simulink model "Rocketmodel"  (R2024b)
settings: Solver=FixedStepDiscrete  StartTime=0.0  StopTime=20  FixedStep=0.001  RelTol=1e-3
values from neighbouring files (symbols this model uses):
  Euler0 = [0 0 -3]/57.3    [Trajectory_Optimization.m]
  Omega0 = [0 0 0]/57.3    [Trajectory_Optimization.m]
  R0 = [36 748 0]    [Trajectory_Optimization.m]
  V0 = [-8.6 -69.6 0]    [Trajectory_Optimization.m]
undefined symbols (not defined in the file or in its folder): den_Engine, den_GZ, den_SF, DiscIntNeverNeededParam, dspblkCoreblockFVToolHelper, Euler, gcbh, num_Engine, num_GZ, num_SF, R, Tc, Ts
libraries: simulink x2
settings Model: Creator=Administrator  LastModifiedBy=Administrator
settings SolverCC: AlgebraicLoopSolver=TrustRegion
settings DebuggingCC: ArithmeticOperatorsInVariantConditions=warning
settings SFSimCC: CustomCodeUndefinedFunction=UseInterfaceOnly
settings RTWCC: GPUComputeCapability=3.5

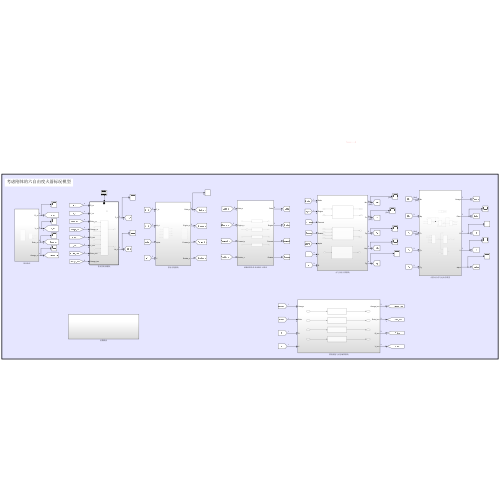
[thumbnail: Simulink's stored preview of the top-level diagram]
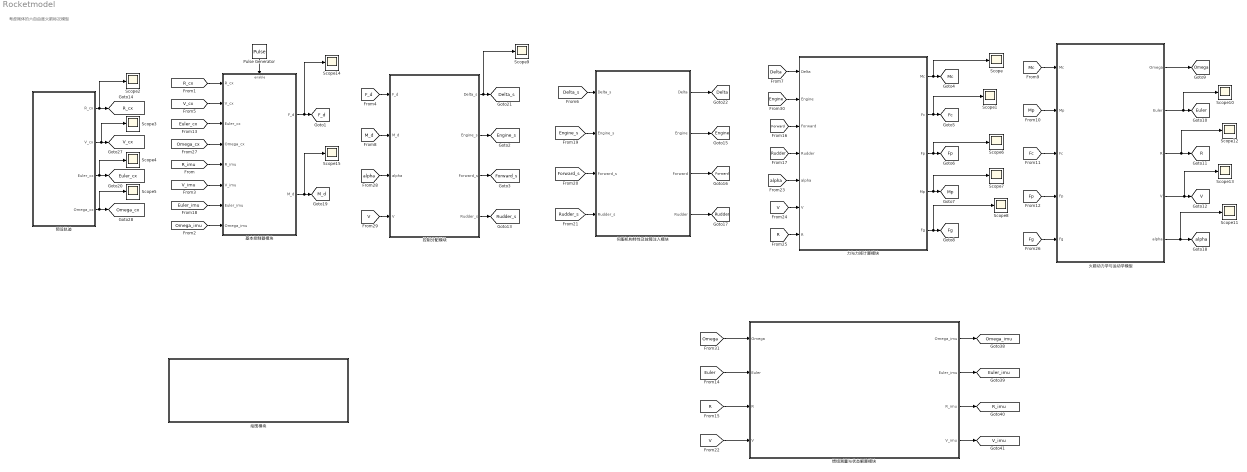
== system Rocketmodel ==
  note: 考虑刚体的六自由度火箭标况模型
  Pulse Generator : DiscretePulseGenerator  Period=Tc/Ts  SampleTime=-1
  Scope{,1..15} (16 alike) : Scope
  伺服机构特性及故障注入模块 : Subsystem
  力与力矩计算模块 : Subsystem
  基本控制器模块 : Subsystem  TreatAsAtomicUnit=on
  惯组测量与状态解算模块 : Subsystem
  控制分配模块 : Subsystem
  火箭动力学与运动学模型 : Subsystem
  绘图模块 : Subsystem
  预设轨迹 : Subsystem
  tag scope: Delta=global, Delta_s=global, Engine=global, Engine_s=global, Euler=global, Euler_cx=global, Euler_imu=global, F_d=global, Fc=global, Fg=global, Forward=global, Forward_s=global, Fp=global, M_d=global, Mc=global, Mp=global, Omega=global, Omega_cx=global, Omega_imu=global, R=global, R_cx=global, R_imu=global, Rudder=global, Rudder_s=global, V=global, V_cx=global, V_imu=global, alpha=global
  wires:
  基本控制器模块/2(M_d) -> Scope15/1, [M_d]
  [Delta_s] -> 伺服机构特性及故障注入模块/1(Delta_s)
  [R_cx] -> 基本控制器模块/1(R_cx)
  Pulse Generator/1 -> 基本控制器模块/Enable
  [R_imu] -> 基本控制器模块/5(R_imu)
  [Euler_imu] -> 基本控制器模块/7(Euler_imu)
  [Omega] -> 惯组测量与状态解算模块/1(Omega)
  惯组测量与状态解算模块/1(Omega_imu) -> [Omega_imu]
  惯组测量与状态解算模块/2(Euler_imu) -> [Euler_imu]
  惯组测量与状态解算模块/3(R_imu) -> [R_imu]
  [Omega_imu] -> 基本控制器模块/8(Omega_imu)
  [V_imu] -> 基本控制器模块/6(V_imu)
  基本控制器模块/1(F_d) -> Scope14/1, [F_d]
  伺服机构特性及故障注入模块/1(Delta) -> [Delta]
  [Engine_s] -> 伺服机构特性及故障注入模块/2(Engine_s)
  [Forward_s] -> 伺服机构特性及故障注入模块/3(Forward_s)
  [Rudder_s] -> 伺服机构特性及故障注入模块/4(Rudder_s)
  伺服机构特性及故障注入模块/4(Rudder) -> [Rudder]
  伺服机构特性及故障注入模块/3(Forward) -> [Forward]
  伺服机构特性及故障注入模块/2(Engine) -> [Engine]
  [Delta] -> 力与力矩计算模块/1(Delta)
  [Engine] -> 力与力矩计算模块/2(Engine)
  [Forward] -> 力与力矩计算模块/3(Forward)
  [Rudder] -> 力与力矩计算模块/4(Rudder)
  力与力矩计算模块/1(Mc) -> Scope/1, [Mc]
  力与力矩计算模块/5(Fg) -> Scope8/1, [Fg]
  力与力矩计算模块/4(Mp) -> Scope7/1, [Mp]
  力与力矩计算模块/3(Fp) -> Scope6/1, [Fp]
  力与力矩计算模块/2(Fc) -> Scope1/1, [Fc]
  [Mc] -> 火箭动力学与运动学模型/1(Mc)
  [Fc] -> 火箭动力学与运动学模型/3(Fc)
  [Fp] -> 火箭动力学与运动学模型/4(Fp)
  [Mp] -> 火箭动力学与运动学模型/2(Mp)
  火箭动力学与运动学模型/1(Omega) -> [Omega]
  火箭动力学与运动学模型/2(Euler) -> Scope10/1, [Euler]
  火箭动力学与运动学模型/3(R) -> Scope12/1, [R]
  火箭动力学与运动学模型/4(V) -> Scope13/1, [V]
  火箭动力学与运动学模型/5(alpha) -> Scope11/1, [alpha]
  [Euler] -> 惯组测量与状态解算模块/2(Euler)
  [R] -> 惯组测量与状态解算模块/3(R)
  [V] -> 惯组测量与状态解算模块/4(V)
  惯组测量与状态解算模块/4(V_imu) -> [V_imu]
  [V] -> 力与力矩计算模块/6(V)
  [R] -> 力与力矩计算模块/7(R)
  [Fg] -> 火箭动力学与运动学模型/5(Fg)
  ? -> ?
  预设轨迹/1(R_cx) -> [R_cx], Scope2/1
  预设轨迹/3(Euler_cx) -> Scope4/1, [Euler_cx]
  预设轨迹/2(V_cx) -> Scope3/1, [V_cx]
  预设轨迹/4(Omega_cx) -> Scope5/1, [Omega_cx]
  [Omega_cx] -> 基本控制器模块/4(Omega_cx)
  [Euler_cx] -> 基本控制器模块/3(Euler_cx)
  [V_cx] -> 基本控制器模块/2(V_cx)
  [alpha] -> 力与力矩计算模块/5(alpha)
  [M_d] -> 控制分配模块/2(M_d)
  控制分配模块/3(Forward_s) -> [Forward_s]
  [F_d] -> 控制分配模块/1(F_d)
  控制分配模块/2(Engine_s) -> [Engine_s]
  控制分配模块/1(Delta_s) -> Scope9/1, [Delta_s]
  控制分配模块/4(Rudder_s) -> [Rudder_s]
  [alpha] -> 控制分配模块/3(alpha)
  [V] -> 控制分配模块/4(V)

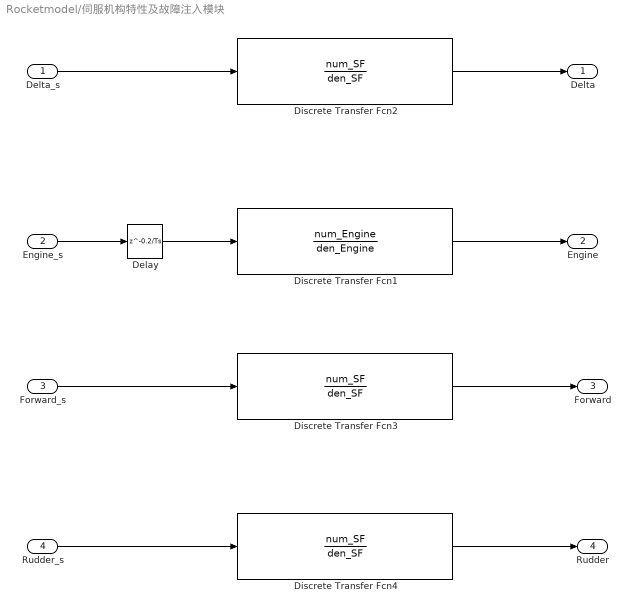
== system Rocketmodel/伺服机构特性及故障注入模块 ==
  Delta_s : Inport
  Engine_s : Inport  Port=2
  Forward_s : Inport  Port=3
  Rudder_s : Inport  Port=4
  Delay : Delay  DelayLength=0.2/Ts  InitialCondition=0
  Discrete Transfer Fcn1 : DiscreteTransferFcn  LoadFcn=dspblkCoreblockFVToolHelper(gcbh,'load');  Numerator=num_Engine  Denominator=den_Engine
      settings: CopyFcn=dspblkCoreblockFVToolHelper(gcbh,'copy');  DeleteFcn=dspblkCoreblockFVToolHelper(gcbh,'close');  ModelCloseFcn=dspblkCoreblockFVToolHelper(gcbh,'close');  PreSaveFcn=dspblkCoreblockFVToolHelper(gcbh,'presave');  PostSaveFcn=dspblkCoreblockFVToolHelper(gcbh,'postsave');  CloseFcn=dspblkCoreblockFVToolHelper(gcbh,'close');
  Discrete Transfer Fcn2 : DiscreteTransferFcn  LoadFcn=dspblkCoreblockFVToolHelper(gcbh,'load');  Numerator=num_SF  Denominator=den_SF
      settings: CopyFcn=dspblkCoreblockFVToolHelper(gcbh,'copy');  DeleteFcn=dspblkCoreblockFVToolHelper(gcbh,'close');  ModelCloseFcn=dspblkCoreblockFVToolHelper(gcbh,'close');  PreSaveFcn=dspblkCoreblockFVToolHelper(gcbh,'presave');  PostSaveFcn=dspblkCoreblockFVToolHelper(gcbh,'postsave');  CloseFcn=dspblkCoreblockFVToolHelper(gcbh,'close');
  Discrete Transfer Fcn3 : DiscreteTransferFcn  LoadFcn=dspblkCoreblockFVToolHelper(gcbh,'load');  Numerator=num_SF  Denominator=den_SF
      settings: CopyFcn=dspblkCoreblockFVToolHelper(gcbh,'copy');  DeleteFcn=dspblkCoreblockFVToolHelper(gcbh,'close');  ModelCloseFcn=dspblkCoreblockFVToolHelper(gcbh,'close');  PreSaveFcn=dspblkCoreblockFVToolHelper(gcbh,'presave');  PostSaveFcn=dspblkCoreblockFVToolHelper(gcbh,'postsave');  CloseFcn=dspblkCoreblockFVToolHelper(gcbh,'close');
  Discrete Transfer Fcn4 : DiscreteTransferFcn  LoadFcn=dspblkCoreblockFVToolHelper(gcbh,'load');  Numerator=num_SF  Denominator=den_SF
      settings: CopyFcn=dspblkCoreblockFVToolHelper(gcbh,'copy');  DeleteFcn=dspblkCoreblockFVToolHelper(gcbh,'close');  ModelCloseFcn=dspblkCoreblockFVToolHelper(gcbh,'close');  PreSaveFcn=dspblkCoreblockFVToolHelper(gcbh,'presave');  PostSaveFcn=dspblkCoreblockFVToolHelper(gcbh,'postsave');  CloseFcn=dspblkCoreblockFVToolHelper(gcbh,'close');
  Delta : Outport
  Engine : Outport  Port=2
  Forward : Outport  Port=3
  Rudder : Outport  Port=4
  wires:
  Delay/1 -> Discrete Transfer Fcn1/1
  Engine_s/1 -> Delay/1
  Delta_s/1 -> Discrete Transfer Fcn2/1
  Forward_s/1 -> Discrete Transfer Fcn3/1
  Rudder_s/1 -> Discrete Transfer Fcn4/1
  Discrete Transfer Fcn2/1 -> Delta/1
  Discrete Transfer Fcn1/1 -> Engine/1
  Discrete Transfer Fcn3/1 -> Forward/1
  Discrete Transfer Fcn4/1 -> Rudder/1

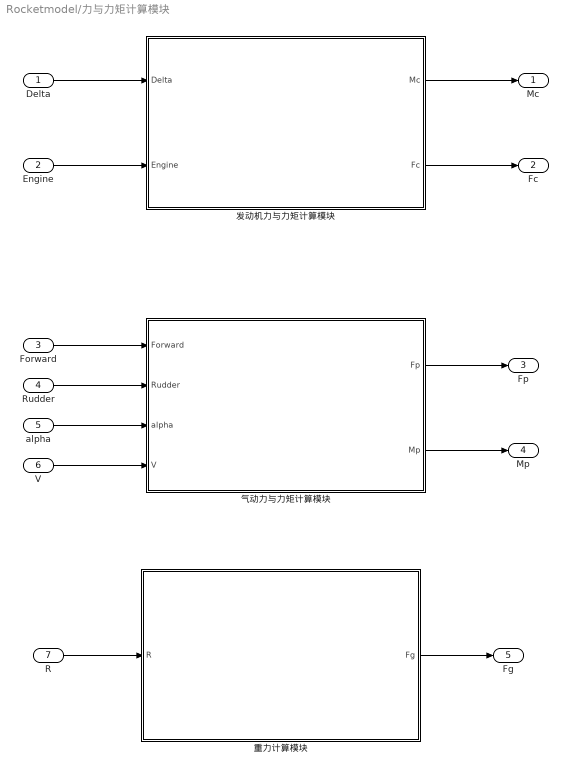
== system Rocketmodel/力与力矩计算模块 ==
  Delta : Inport
  Engine : Inport  Port=2
  Forward : Inport  Port=3
  Rudder : Inport  Port=4
  alpha : Inport  Port=5
  V : Inport  Port=6
  R : Inport  Port=7
  发动机力与力矩计算模块 : Subsystem
  气动力与力矩计算模块 : Subsystem
  重力计算模块 : Subsystem
  Mc : Outport
  Fc : Outport  Port=2
  Fp : Outport  Port=3
  Mp : Outport  Port=4
  Fg : Outport  Port=5
  wires:
  发动机力与力矩计算模块/2(Fc) -> Fc/1
  发动机力与力矩计算模块/1(Mc) -> Mc/1
  Delta/1 -> 发动机力与力矩计算模块/1(Delta)
  Engine/1 -> 发动机力与力矩计算模块/2(Engine)
  Forward/1 -> 气动力与力矩计算模块/1(Forward)
  Rudder/1 -> 气动力与力矩计算模块/2(Rudder)
  alpha/1 -> 气动力与力矩计算模块/3(alpha)
  V/1 -> 气动力与力矩计算模块/4(V)
  气动力与力矩计算模块/2(Mp) -> Mp/1
  气动力与力矩计算模块/1(Fp) -> Fp/1
  R/1 -> 重力计算模块/1(R)
  重力计算模块/1(Fg) -> Fg/1

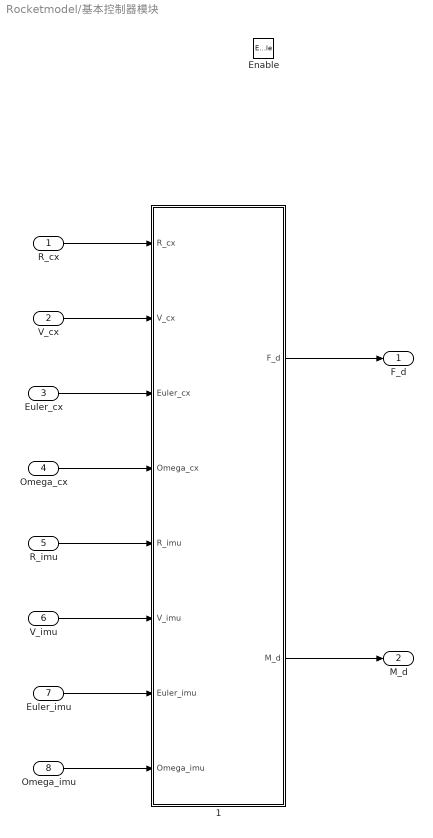
== system Rocketmodel/基本控制器模块 ==
  R_cx : Inport
  V_cx : Inport  Port=2
  Euler_cx : Inport  Port=3
  Omega_cx : Inport  Port=4
  R_imu : Inport  Port=5
  V_imu : Inport  Port=6
  Euler_imu : Inport  Port=7
  Omega_imu : Inport  Port=8
  Enable : EnablePort
  1 : MATLAB Function  TreatAsAtomicUnit=on
  F_d : Outport
  M_d : Outport  Port=2
  wires:
  R_cx/1 -> 1/1(R_cx)
  R_imu/1 -> 1/5(R_imu)
  V_imu/1 -> 1/6(V_imu)
  Euler_imu/1 -> 1/7(Euler_imu)
  Omega_imu/1 -> 1/8(Omega_imu)
  1/1(F_d) -> F_d/1
  V_cx/1 -> 1/2(V_cx)
  Euler_cx/1 -> 1/3(Euler_cx)
  Omega_cx/1 -> 1/4(Omega_cx)
  1/2(M_d) -> M_d/1

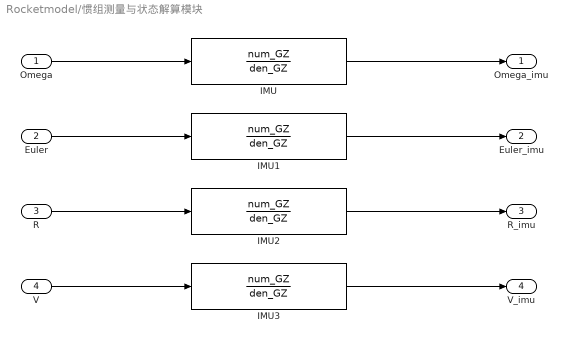
== system Rocketmodel/惯组测量与状态解算模块 ==
  Omega : Inport
  Euler : Inport  Port=2
  R : Inport  Port=3
  V : Inport  Port=4
  IMU{,1..3} (4 alike) : DiscreteTransferFcn  LoadFcn=dspblkCoreblockFVToolHelper(gcbh,'load');  Numerator=num_GZ  Denominator=den_GZ
      settings: CopyFcn=dspblkCoreblockFVToolHelper(gcbh,'copy');  DeleteFcn=dspblkCoreblockFVToolHelper(gcbh,'close');  ModelCloseFcn=dspblkCoreblockFVToolHelper(gcbh,'close');  PreSaveFcn=dspblkCoreblockFVToolHelper(gcbh,'presave');  PostSaveFcn=dspblkCoreblockFVToolHelper(gcbh,'postsave');  CloseFcn=dspblkCoreblockFVToolHelper(gcbh,'close');
  Omega_imu : Outport
  Euler_imu : Outport  Port=2
  R_imu : Outport  Port=3
  V_imu : Outport  Port=4
  wires:
  IMU/1 -> Omega_imu/1
  Omega/1 -> IMU/1
  IMU3/1 -> V_imu/1
  IMU2/1 -> R_imu/1
  IMU1/1 -> Euler_imu/1
  Euler/1 -> IMU1/1
  R/1 -> IMU2/1
  V/1 -> IMU3/1

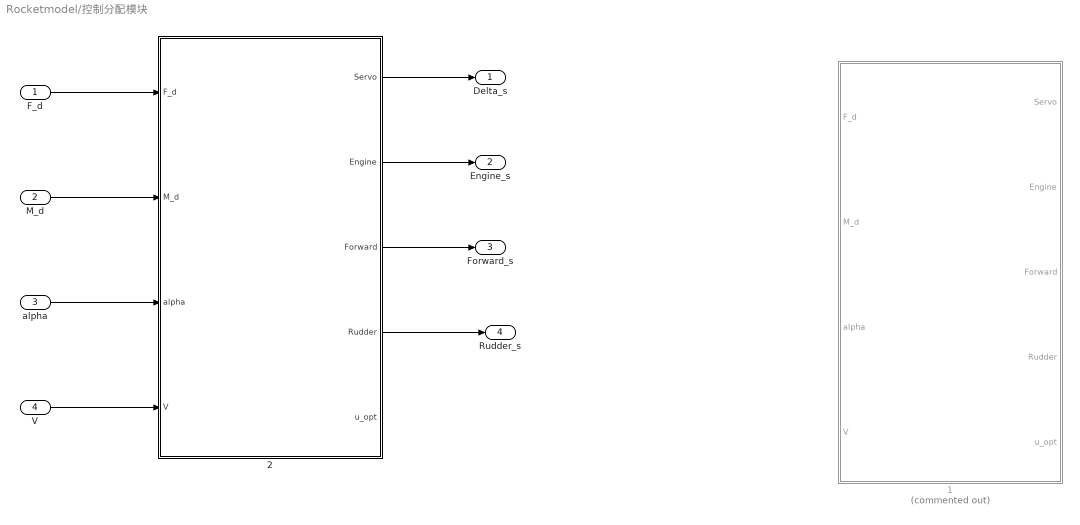
== system Rocketmodel/控制分配模块 ==
  F_d : Inport
  M_d : Inport  Port=2
  alpha : Inport  Port=3
  V : Inport  Port=4
  1 : MATLAB Function  Commented=on  TreatAsAtomicUnit=on
  2 : MATLAB Function  TreatAsAtomicUnit=on
  Delta_s : Outport
  Engine_s : Outport  Port=2
  Forward_s : Outport  Port=3
  Rudder_s : Outport  Port=4
  wires:
  2/1(Servo) -> Delta_s/1
  2/2(Engine) -> Engine_s/1
  2/3(Forward) -> Forward_s/1
  2/4(Rudder) -> Rudder_s/1
  F_d/1 -> 2/1(F_d)
  M_d/1 -> 2/2(M_d)
  alpha/1 -> 2/3(alpha)
  V/1 -> 2/4(V)

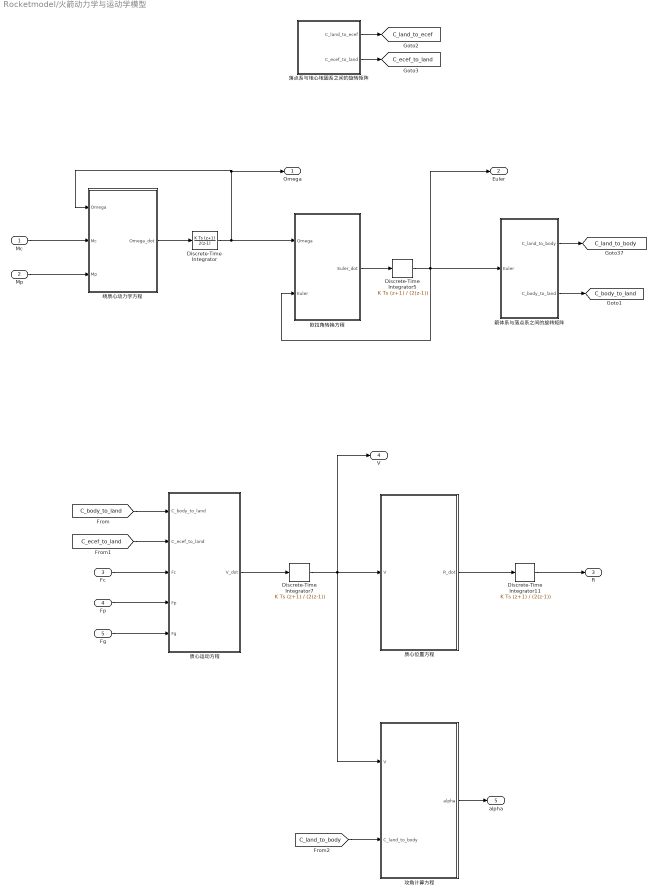
== system Rocketmodel/火箭动力学与运动学模型 ==
  Mc : Inport
  Mp : Inport  Port=2
  Fc : Inport  Port=3
  Fp : Inport  Port=4
  Fg : Inport  Port=5
  Discrete-Time Integrator : DiscreteIntegrator  IntegratorMethod=Integration: Trapezoidal  InitialCondition=Omega0  SampleTime=-1  ICPrevOutput=DiscIntNeverNeededParam  ICPrevScaledInput=DiscIntNeverNeededParam
  Discrete-Time Integrator11 : DiscreteIntegrator  IntegratorMethod=Integration: Trapezoidal  InitialCondition=R0  SampleTime=-1  ICPrevOutput=DiscIntNeverNeededParam  ICPrevScaledInput=DiscIntNeverNeededParam
  Discrete-Time Integrator5 : DiscreteIntegrator  IntegratorMethod=Integration: Trapezoidal  InitialCondition=Euler0  SampleTime=-1  ICPrevOutput=DiscIntNeverNeededParam  ICPrevScaledInput=DiscIntNeverNeededParam
  Discrete-Time Integrator7 : DiscreteIntegrator  IntegratorMethod=Integration: Trapezoidal  InitialCondition=V0  SampleTime=-1  ICPrevOutput=DiscIntNeverNeededParam  ICPrevScaledInput=DiscIntNeverNeededParam
  攻角计算方程 : MATLAB Function  TreatAsAtomicUnit=on
  欧拉角转换方程 : MATLAB Function  TreatAsAtomicUnit=on
  箭体系与落点系之间的旋转矩阵 : MATLAB Function  TreatAsAtomicUnit=on
  绕质心动力学方程 : MATLAB Function  TreatAsAtomicUnit=on
  落点系与地心地固系之间的旋转矩阵 : MATLAB Function  TreatAsAtomicUnit=on
  质心位置方程 : MATLAB Function  TreatAsAtomicUnit=on
  质心运动方程 : MATLAB Function  TreatAsAtomicUnit=on
  Omega : Outport
  Euler : Outport  Port=2
  R : Outport  Port=3
  V : Outport  Port=4
  alpha : Outport  Port=5
  tag scope: C_body_to_land=global, C_ecef_to_land=global, C_land_to_body=global, C_land_to_ecef=global
  wires:
  Fp/1 -> 质心运动方程/4(Fp)
  Mc/1 -> 绕质心动力学方程/2(Mc)
  绕质心动力学方程/1(Omega_dot) -> Discrete-Time Integrator/1
  质心位置方程/1(R_dot) -> Discrete-Time Integrator11/1
  落点系与地心地固系之间的旋转矩阵/2(C_ecef_to_land) -> [C_ecef_to_land]
  质心运动方程/1(V_dot) -> Discrete-Time Integrator7/1
  [C_body_to_land] -> 质心运动方程/1(C_body_to_land)
  Discrete-Time Integrator5/1 -> Euler/1, 箭体系与落点系之间的旋转矩阵/1(Euler), 欧拉角转换方程/2(Euler)
  Mp/1 -> 绕质心动力学方程/3(Mp)
  落点系与地心地固系之间的旋转矩阵/1(C_land_to_ecef) -> [C_land_to_ecef]
  Fg/1 -> 质心运动方程/5(Fg)
  Discrete-Time Integrator7/1 -> 攻角计算方程/1(V), V/1, 质心位置方程/1(V)
  Discrete-Time Integrator/1 -> 欧拉角转换方程/1(Omega), 绕质心动力学方程/1(Omega), Omega/1
  [C_ecef_to_land] -> 质心运动方程/2(C_ecef_to_land)
  箭体系与落点系之间的旋转矩阵/1(C_land_to_body) -> [C_land_to_body]
  Discrete-Time Integrator11/1 -> R/1
  欧拉角转换方程/1(Euler_dot) -> Discrete-Time Integrator5/1
  攻角计算方程/1(alpha) -> alpha/1
  Fc/1 -> 质心运动方程/3(Fc)
  [C_land_to_body] -> 攻角计算方程/2(C_land_to_body)
  箭体系与落点系之间的旋转矩阵/2(C_body_to_land) -> [C_body_to_land]

== system Rocketmodel/绘图模块 ==

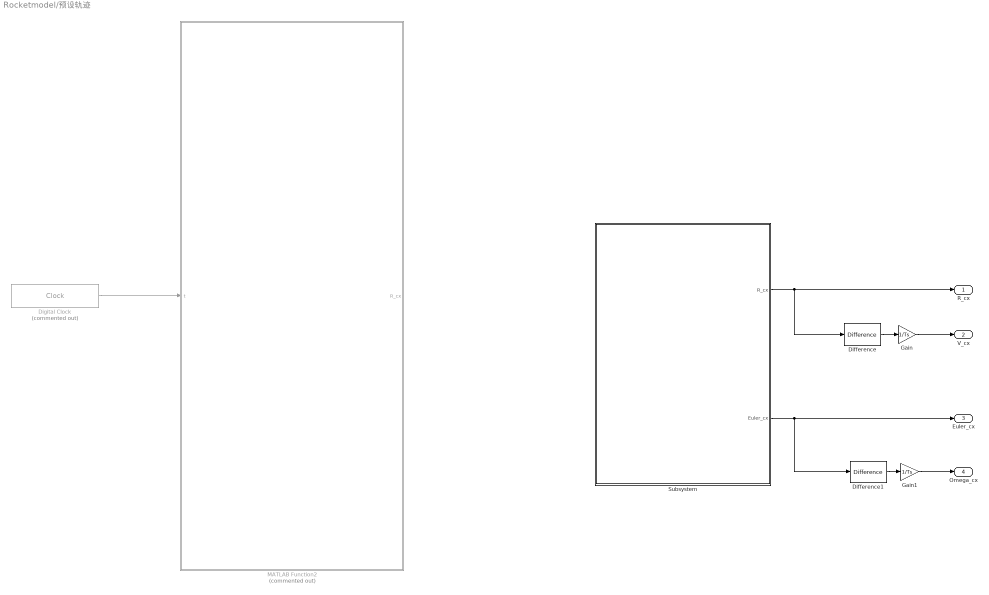
== system Rocketmodel/预设轨迹 ==
  Difference : simulink/Discrete/Difference  ICPrevInput=R(:,1)  OutMin=[]  OutMax=[]  OutDataType=fixdt(1, 16)  OutScaling=2^-10  DoSatur=off
  Difference1 : simulink/Discrete/Difference  ICPrevInput=Euler(:,1)  OutMin=[]  OutMax=[]  OutDataType=fixdt(1, 16)  OutScaling=2^-10  DoSatur=off
  Digital Clock : DigitalClock  Commented=on  SampleTime=Ts
  Gain : Gain  Gain=1/Ts
  Gain1 : Gain  Gain=1/Ts
  MATLAB Function2 : MATLAB Function  Commented=on  TreatAsAtomicUnit=on
  Subsystem : Subsystem
  R_cx : Outport
  V_cx : Outport  Port=2
  Euler_cx : Outport  Port=3
  Omega_cx : Outport  Port=4
  wires:
  Digital Clock/1 -> MATLAB Function2/1(t)
  Difference/1 -> Gain/1
  Difference1/1 -> Gain1/1
  Subsystem/1(R_cx) -> Difference/1, R_cx/1
  Subsystem/2(Euler_cx) -> Difference1/1, Euler_cx/1
  Gain/1 -> V_cx/1
  Gain1/1 -> Omega_cx/1

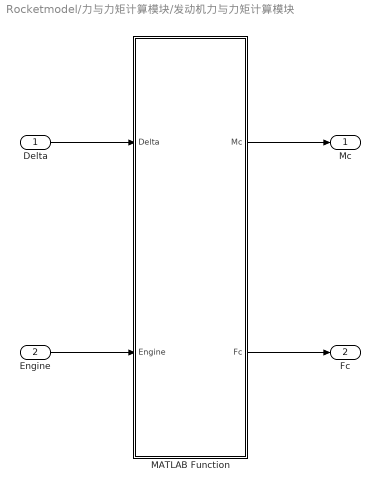
== system Rocketmodel/力与力矩计算模块/发动机力与力矩计算模块 ==
  Delta : Inport
  Engine : Inport  Port=2
  MATLAB Function : MATLAB Function  TreatAsAtomicUnit=on
  Mc : Outport
  Fc : Outport  Port=2
  wires:
  MATLAB Function/1(Mc) -> Mc/1
  MATLAB Function/2(Fc) -> Fc/1
  Delta/1 -> MATLAB Function/1(Delta)
  Engine/1 -> MATLAB Function/2(Engine)

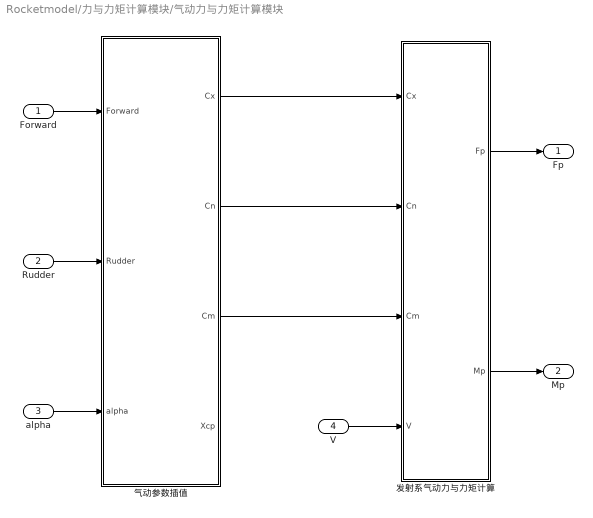
== system Rocketmodel/力与力矩计算模块/气动力与力矩计算模块 ==
  Forward : Inport
  Rudder : Inport  Port=2
  alpha : Inport  Port=3
  V : Inport  Port=4
  发射系气动力与力矩计算 : MATLAB Function  TreatAsAtomicUnit=on
  气动参数插值 : MATLAB Function  TreatAsAtomicUnit=on
  Fp : Outport
  Mp : Outport  Port=2
  wires:
  发射系气动力与力矩计算/1(Fp) -> Fp/1
  发射系气动力与力矩计算/2(Mp) -> Mp/1
  V/1 -> 发射系气动力与力矩计算/4(V)
  Forward/1 -> 气动参数插值/1(Forward)
  Rudder/1 -> 气动参数插值/2(Rudder)
  alpha/1 -> 气动参数插值/3(alpha)
  气动参数插值/1(Cx) -> 发射系气动力与力矩计算/1(Cx)
  气动参数插值/2(Cn) -> 发射系气动力与力矩计算/2(Cn)
  气动参数插值/3(Cm) -> 发射系气动力与力矩计算/3(Cm)

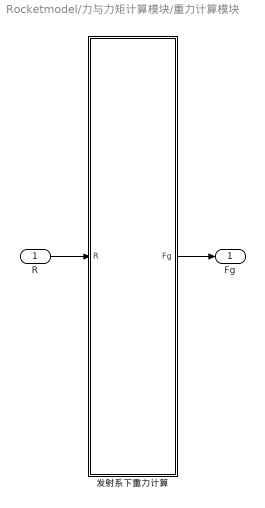
== system Rocketmodel/力与力矩计算模块/重力计算模块 ==
  R : Inport
  发射系下重力计算 : MATLAB Function  TreatAsAtomicUnit=on
  Fg : Outport
  wires:
  发射系下重力计算/1(Fg) -> Fg/1
  R/1 -> 发射系下重力计算/1(R)

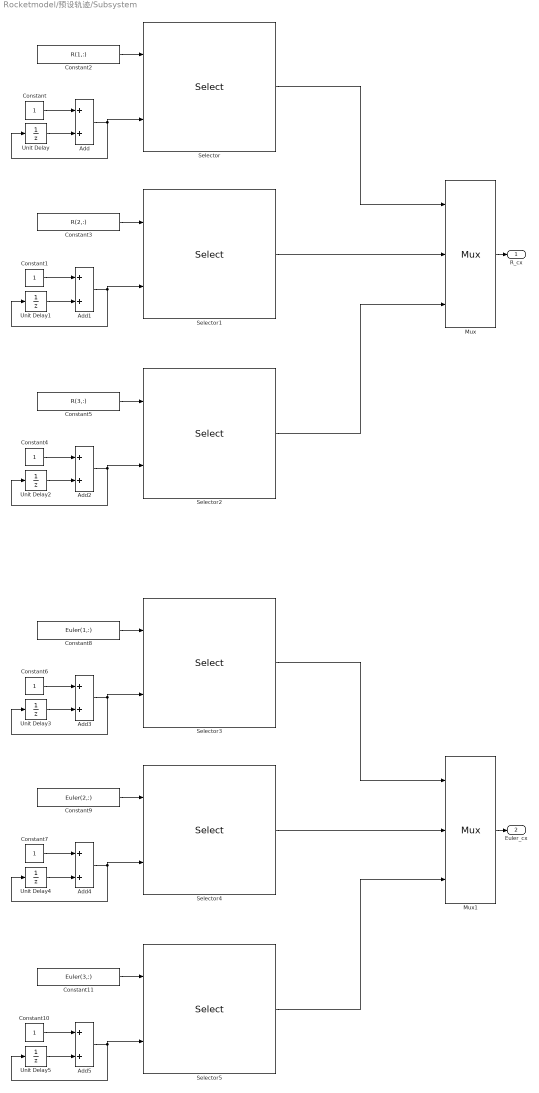
== system Rocketmodel/预设轨迹/Subsystem ==
  Add{,1..5} (6 alike) : Sum
  Constant{,1,4,6..7,10} (6 alike) : Constant
  Constant11 : Constant  Value=Euler(3,:)
  Constant2 : Constant  Value=R(1,:)
  Constant3 : Constant  Value=R(2,:)
  Constant5 : Constant  Value=R(3,:)
  Constant8 : Constant  Value=Euler(1,:)
  Constant9 : Constant  Value=Euler(2,:)
  Mux : Mux  Inputs=3
  Mux1 : Mux  Inputs=3
  Selector{,1..5} (6 alike) : Selector  InputPortWidth=20001  IndexOptions=Index vector (port)  Indices=[1 3]  OutputSizes=1
  Unit Delay{,1..5} (6 alike) : UnitDelay  SampleTime=-1  HasFrameUpgradeWarning=on
  R_cx : Outport
  Euler_cx : Outport  Port=2
  wires:
  Unit Delay/1 -> Add/2
  Constant/1 -> Add/1
  Add/1 -> Unit Delay/1, Selector/2
  Constant2/1 -> Selector/1
  Add1/1 -> Unit Delay1/1, Selector1/2
  Unit Delay1/1 -> Add1/2
  Constant3/1 -> Selector1/1
  Constant1/1 -> Add1/1
  Add2/1 -> Unit Delay2/1, Selector2/2
  Unit Delay2/1 -> Add2/2
  Constant5/1 -> Selector2/1
  Constant4/1 -> Add2/1
  Selector1/1 -> Mux/2
  Selector/1 -> Mux/1
  Selector2/1 -> Mux/3
  Mux/1 -> R_cx/1
  Unit Delay3/1 -> Add3/2
  Constant8/1 -> Selector3/1
  Constant6/1 -> Add3/1
  Unit Delay5/1 -> Add5/2
  Constant10/1 -> Add5/1
  Add5/1 -> Unit Delay5/1, Selector5/2
  Unit Delay4/1 -> Add4/2
  Add4/1 -> Unit Delay4/1, Selector4/2
  Constant7/1 -> Add4/1
  Constant11/1 -> Selector5/1
  Selector4/1 -> Mux1/2
  Mux1/1 -> Euler_cx/1
  Constant9/1 -> Selector4/1
  Selector3/1 -> Mux1/1
  Add3/1 -> Unit Delay3/1, Selector3/2
  Selector5/1 -> Mux1/3

== matlab function Rocketmodel/预设轨迹/MATLAB Function2 ==
  data: R_cx output; t input
function R_cx  = fcn(t)

% 初始位置、速度
R0 = [36 748 0]';
V0 = [-8.6 -69.6 0]';

%目标位置、速度
R1 = [0 0 0]';
V1 = [0 0 0]';

% 初始欧拉角、欧拉角速度
Euler0 = [0 0 -3]'/57.3;
Omega0 = [0 0 0]'/57.3;

% 目标欧拉角、欧拉角速度
Euler1 = [0 0 90]'/57.3;
Omega1 = [0 0 0]'/57.3;


% 1. 时间定义
Ts = 0.001;
T_flip = 5;        % 翻转阶段时间
T_land = 15;       % 垂直下降阶段时间

T_flip = 0:Ts:T_flip;
T_land = Ts:Ts:T_land;
T = [T_flip T_flip(end)+T_land]; % 总时间

% 2. 初始状态

phi1 = 90/57.3; psi1 = 0; gamma1 = 0; % 目标姿态(rad)

% 3. 阶段1 翻转
% 姿态
N_flip = length(T_flip);
phi_flip = linspace(Euler0(3), Euler1(3), N_flip);  % φ
psi_flip = linspace(Euler0(2), Euler1(2), N_flip);  % ψ
gamma_flip = linspace(Euler0(1), Euler1(1), N_flip); % γ

% 位置
R_flip = zeros(3,N_flip);
R_flip(1,:) = R0(1) + V0(1)*T_flip;
R_flip(2,:) = R0(2) + V0(2)*T_flip - 0.5*9.81*T_flip.^2;
R_flip(3,:) = R0(3) + V0(3)*T_flip;

% 4. 阶段2 垂直下降
N_land = length(T_land);
phi_land = ones(1,N_land)*phi1;
psi_land = ones(1,N_land)*psi1;
gamma_land = ones(1,N_land)*gamma1;

R_land = zeros(3,N_land);
R_land(1,:) = linspace(R_flip(1,end), R1(1), N_land);
R_land(2,:) = linspace(R_flip(2,end), R1(2), N_land);
R_land(3,:) = linspace(R_flip(3,end), R1(3), N_land);

% 5. 合并
R = [R_flip R_land];           % 3xN
Euler = [gamma_flip; psi_flip; phi_flip];
Euler = [Euler [gamma_land; psi_land; phi_land]];

R_cx = R(:,(t+1)/Ts);

== matlab function Rocketmodel/基本控制器模块/1 ==
  data: F_d output; R_cx input; V_cx input; Euler_cx input; Omega_cx input; R_imu input; V_imu input; Euler_imu input; Omega_imu input; M_d output
function [F_d, M_d]= allocation(R_cx,V_cx,Euler_cx, Omega_cx,R_imu,V_imu, Euler_imu, Omega_imu)

%% 函数说明

% 在控制周期内，根据位置、速度、欧拉角、角速度目标值与测量值，计算得到三通道期望力、期望力矩





%% 基本参数引入

M0 = 155975;                     % 火箭质量
I = diag([194500, 13280000,13280000]);        % 惯性矩阵

% Kp_pos = 1;  Kd_pos = 0;
% Kp_att = 1; Kd_att = 0;

Kp_pos = [0 0 0;0 0 0;0 0 0];  
Kd_pos =[0 0 0;0 0 0;0 0 0];  

Kp_att = [0 0 0;0 0 0;0 0 1];

Kd_att = [0 0 0;0 0 0;0 0 0.5];  



%% 转换矩阵（机体系与落点系）
C_land_to_body = [cos(Euler_imu(3)) * cos(Euler_imu(2)), sin(Euler_imu(3)) * cos(Euler_imu(2)), - sin(Euler_imu(2));
    - sin(Euler_imu(3))*cos(Euler_imu(1)) + cos(Euler_imu(3))*sin(Euler_imu(2))*sin(Euler_imu(1)), cos(Euler_imu(3))*cos(Euler_imu(1)) + sin(Euler_imu(3))*sin(Euler_imu(2))*sin(Euler_imu(1)), cos(Euler_imu(2))*sin(Euler_imu(1));
    sin(Euler_imu(3))*sin(Euler_imu(1)) + cos(Euler_imu(3))*sin(Euler_imu(2))*cos(Euler_imu(1)), - cos(Euler_imu(3))*sin(Euler_imu(1)) + sin(Euler_imu(3))*sin(Euler_imu(2))*cos(Euler_imu(1)), cos(Euler_imu(2))*cos(Euler_imu(1))];

C_body_to_land =  C_land_to_body'; 

%% --- 落点系下的平移控制 ---

e_R = R_cx - R_imu;          % 位置误差 (落点系)
e_V = V_cx - V_imu;          % 速度误差 (落点系)

a_d = Kp_pos*e_R + Kd_pos*e_V;  % 期望加速度 (落点系)
F_d = M0 * a_d;                  % 期望力 (落点系)

F_d = C_land_to_body * F_d;                  % 期望力 (机体系)

%% --- 机体系下的姿态控制 ---

% 姿态误差 
e_Euler = Euler_cx - Euler_imu;

% 角速度误差 (机体系)
e_Omega = Omega_cx - Omega_imu;

% 控制律得到期望角加速度 (机体系)
alpha_d = Kp_att*e_Euler + Kd_att*e_Omega;

% 惯性矩阵映射到期望力矩 (机体系)
M_d = I * alpha_d;



end

== matlab function Rocketmodel/控制分配模块/2 ==
  data: Servo output; F_d input; M_d input; alpha input; Engine output; Forward output; Rudder output; u_opt output; V input
function [Servo, Engine, Forward, Rudder, u_opt] = allocation_opt(F_d, M_d, alpha, V)


persistent u_prev  % 保存上一时刻优化解
%% ================== 初始猜测 ==================
% 第一次调用时初始化
if isempty(u_prev)
    u_prev = zeros(9,1);  % 必须先给值
end

% 初始猜测使用上一时刻解
u0 = u_prev;


%% ================== 内部参数定义 ==================
N_engine = 3;  % 发动机数量
Pe = 2.45e6;   % 单台发动机额定推力 [N]
r_engine = [ -15.2740  -15.2740  -15.2740;
               1.5      -0.75     -0.75;
               0        -1.299     1.299 ];  % 发动机在机体系下位置 [m]

%% ================== 单变量上下界 ==================
lb = [-7.8*pi/180*ones(6,1); zeros(3,1)];
ub = [ 7.8*pi/180*ones(6,1); ones(3,1)];

%% ================== 等式约束、力矩配平 ==================
A_eq = zeros(3,9);
b_eq = zeros(3,1);
A_eq(2)=1;
A_eq(4)=1;
A_eq(6)=1;

%% ================== 优化器调用 ==================
fun = @(u) cost_function(u, F_d, M_d, N_engine, Pe, r_engine);
options = optimoptions('fmincon','Display','none','Algorithm','sqp', ...
                       'MaxIterations',1000,'OptimalityTolerance',1e-4);
u_opt = fmincon(fun, u0, [], [], A_eq, b_eq, lb, ub, [], options);

% 保存本次解
u_prev = u_opt;

%% ================== 输出拆解 ==================
Servo   = u_opt(1:6);   % 六个伺服角
Engine  = u_opt(7:9);   % 三台发动机推力百分比
Forward = 0;    % 前舵角
Rudder  = 0;    % 后舵角
end


%% ---------------------- 子函数 ----------------------

function J = cost_function(u, F_d, M_d, N_engine, Pe, r_engine)
[F, M] = actuator_model(u, N_engine, Pe, r_engine);
J = norm(F - F_d)^2 + norm(M - M_d)^2;
end

function [F_total, M_total] = actuator_model(u, N_engine, Pe, r_engine)
delta_eng = u(1:6);   % 六个舵机角
P         = u(7:9);   % 三个发动机推力百分比

F_total = zeros(3,1);
M_total = zeros(3,1);

% ================== 三台发动机 ==================
for i = 1:N_engine
    delta_p = delta_eng(2*i-1);
    delta_y = delta_eng(2*i);
    D = [cos(delta_p)*cos(delta_y);
         -sin(delta_p);
         cos(delta_p)*sin(-delta_y)];
    F_i = P(i)*Pe * D;
    M_i = cross(r_engine(:,i), F_i);
    F_total = F_total + F_i;
    M_total = M_total + M_i;
end

end

== matlab function Rocketmodel/力与力矩计算模块/气动力与力矩计算模块/发射系气动力与力矩计算 ==
  data: Fp output; Cx input; Cn input; Cm input; V input; Mp output
function [Fp, Mp] = fcn(Cx, Cn, Cm, V)

%% 函数说明
% 该模块计算箭体系下气动力提供的力与力矩
% 输入参数：
%   气动参数
%   V：箭体系相对于与落点系的速度矢量
% 输出参数：
%   Mp：箭体系下三轴气动力矩 3*1 
%   Fp：箭体系下三轴气动力   3*1


%% 基本参数引入

% 大气密度
pho = 1.2;

% 气动参数面积
S = 63.617;

% 质心与火箭头部的距离
Xz = 28;

% 火箭全长
L = 47.8;

%% 气动力与力矩计算

% 箭体系下气动力计算
Fp = 0.5*pho*norm(V)^2*S*[-Cx, Cn, 0]';

% 箭体系下气动力矩计算
Mp = 0.5*pho*norm(V)^2*S*[0, 0, Cn*Xz - Cm*L]';


end

== matlab function Rocketmodel/力与力矩计算模块/发动机力与力矩计算模块/MATLAB Function ==
  data: Delta input; Mc output; Engine input; Fc output
function [Mc, Fc] = fcn(Delta, Engine)

%% 函数说明
% 该模块计算箭体系下发动机提供的力与力矩
% 输入参数：
%   Delta：发动机摆角 6*1
%   Engine：发动机推力百分比 3*1
% 输出参数：
%   Mc：箭体系下三轴控制力矩 3*1 
%   Fc：箭体系下三轴控制力   3*1

%% 布局参数引入 

% 箭体系下发动机推力作用点位置

R1 = [-15.2740, 1.5, 0]';
R2 = [-15.2740, -0.75, -1.299]';
R3 = [-15.2740, -0.75, 1.299]';

% 单台发动机额定推力

Pe = 2450000;

%% 箭体系下三台发动机力的方向单位向量计算(转序先Y后Z)

D1 = [cos(Delta(1))*cos(Delta(2)), sin(-Delta(1)), cos(Delta(1))*sin(-Delta(2))]';
D2 = [cos(Delta(3))*cos(Delta(4)), sin(-Delta(3)), cos(Delta(3))*sin(-Delta(4))]';
D3 = [cos(Delta(5))*cos(Delta(6)), sin(-Delta(5)), cos(Delta(5))*sin(-Delta(6))]';


%% 箭体系下三台发动机各自力计算

Fc_1 = D1*Pe*Engine(1);
Fc_2 = D2*Pe*Engine(2);
Fc_3 = D3*Pe*Engine(3);


%% 箭体系下三台发动机各自力矩计算

Mc_1 = cross(R1, Fc_1);
Mc_2 = cross(R2, Fc_2);
Mc_3 = cross(R3, Fc_3);


%% 箭体系下三台发动机合力、合力矩计算

Fc = Fc_1 + Fc_2 + Fc_3;
Mc = Mc_1 + Mc_2 + Mc_3;


end

== matlab function Rocketmodel/力与力矩计算模块/重力计算模块/发射系下重力计算 ==
  data: Fg output; R input
function Fg  = fcn(R)

%% 函数说明
% 该模块计算当前火箭在地心地固系下的重力
% 输入参数：
%   R：火箭在地心地固系下的位置
% 输出参数：
%   Fg： 地心地固系下重力 

%%  旋转矩阵、平动向量等参数计算

% 火箭质量

M0 = 155975;

% WGS-84参数

a = 6378137;  
f = 1/298.257223563;
e_2 =2*f - f^2;
b = a*(1 - f);
miu = 3.986004418e14;
J_2 = 1.08263e-3;

% 求落点系land原点在地心地固系ECEF下坐标 
 
L0 = 110.95; %  着陆点经纬高
B0 = 19.6; 
H0 = 0; 

N_B = a/sqrt(1 - e_2*(sind(B0))^2); 
R0_ecef = [(N_B + H0)*cosd(B0)*cosd(L0), (N_B + H0)*cosd(B0)*sind(L0), ((1-e_2)*N_B + H0)*sind(B0)]';


% 求落点系到局部东北天坐标系的旋转矩阵

A0 = 110.3; % 着陆方位角   注意rot函数正数代表顺时针旋转。耽误我好久，气死我了

C_land_to_enu = rotz(90-A0) * rotx(90); 


% 求局部东北天坐标系到地心地固坐标系的旋转矩阵

C_enu_to_ecef = rotz(90+L0)*rotx(90-B0); 

% 求落点系到地心地固系的旋转矩阵 

C_land_to_ecef = C_enu_to_ecef * C_land_to_enu; 

% 求发射系到地心地固系的转换公式 旋转+平动

C_land_to_ecef  = C_land_to_ecef; 
R0_ecef = R0_ecef;



%%  坐标转换 (将落点系下位置转换到地心地固系下位置)

R_ecef = C_land_to_ecef * R + R0_ecef;
x_ECEF = R_ecef(1); 
y_ECEF = R_ecef(2); 
z_ECEF = R_ecef(3); 

%% 地心地固系下重力计算
 
g_ecef = [-miu/(norm(R_ecef))^3*R_ecef(1)*(1-3/2*J_2*(a/norm(R_ecef))^2*(5*(R_ecef(3))^2/(norm(R_ecef))^2 -1)); 
          -miu/(norm(R_ecef))^3*R_ecef(2)*(1-3/2*J_2*(a/norm(R_ecef))^2*(5*(R_ecef(3))^2/(norm(R_ecef))^2 -1));
           -miu/(norm(R_ecef))^3*R_ecef(3)*(1-3/2*J_2*(a/norm(R_ecef))^2*(5*(R_ecef(3))^2/(norm(R_ecef))^2 -3))];


Fg = M0*g_ecef;


end

== matlab function Rocketmodel/力与力矩计算模块/气动力与力矩计算模块/气动参数插值 ==
  data: Cx output; Forward input; Rudder input; alpha input; Cn output; Cm output; Xcp output
function [Cx, Cn, Cm, Xcp]  = fcn(Forward, Rudder, alpha)

%% 函数说明
% 该模块计算当前攻角、前舵角、后舵角下的气动参数
% 输入参数：
%   Forward：前舵舵角
%   Rudder：后舵舵角
%   alpha：攻角
% 输出参数：
%   总的气动参数 4*1 


%% 数据拟合

%================= 基础数据 =================
x = [0,4,8,30,50,60,70,90,150]/57.3;   % 攻角
y = [0,20,40,60,80]/57.3;              % 舵角

% ----------- 前舵数据 -----------------
z_f = [0.2983	0.3105	0.3109	0.34	0.3102	0.36	0.3968	0.3115	-1.178;
0.0333	0.6536	1.442	5.3229	7.9765	8.5087	9.1668	9.894	3.4019;
0.0004	0.3464	0.8089	3.1887	4.5519	4.9497	5.3774	6.0923	2.8019;
0.0126	0.53	0.5609	0.599	0.5707	0.5817	0.5866	0.6158	0.8236;
0.2965	0.3117	0.3068	0.3731	0.3353	0.3577	0.4056	0.3175	-1.1556;
0.0433	0.6561	1.4587	5.4398	7.9116	8.4858	9.1227	9.8364	3.4092;
-0.0002	0.3129	0.7542	3.1904	4.5143	4.9434	5.3699	6.0813	2.8162;
-0.0044	0.4769	0.517	0.5865	0.5706	0.5826	0.5886	0.6182	0.8261;
0.2922	0.3164	0.3073	0.3742	0.3142	0.3435	0.3922	0.3478	-1.1666;
0.0595	0.6854	1.5233	5.6129	8.1435	8.7701	9.4561	10.1558	3.6688;
0.0169	0.3286	0.7791	3.2016	4.5616	4.985	5.4273	6.1567	2.9435;
0.2844	0.4794	0.5114	0.5704	0.5602	0.5684	0.5739	0.6062	0.8023;
0.2862	0.3039	0.2954	0.3019	0.3771	0.3267	0.4269	0.3565	-1.1929;
0.0006	0.6651	1.5116	6.0214	8.2621	9.098	9.5941	10.405	3.7881;
-0.0185	0.3289	0.7783	3.4086	4.5714	5.0651	5.4516	6.2152	2.9431;
0	0.4945	0.5149	0.5661	0.5533	0.5567	0.5682	0.5973	0.7769;
0.242	0.2554	0.2475	0.2483	0.3807	0.3942	0.4246	0.3628	-1.1474;
-0.0001	0.6199	1.4786	6.4426	8.5527	9.1594	9.8809	10.7777	4.0663;
-0.0002	0.29	0.7364	3.7257	4.6952	5.0971	5.57	6.3597	3.0003;
1.9663	0.4678	0.4981	0.5783	0.549	0.5565	0.5637	0.5901	0.7378;
];

% ----------- 后舵数据 -----------------
z_r = [0.242	0.2554	0.2475	0.2483	0.3807	0.3942	0.4246	0.3628	-1.1474;
-0.0001	0.6199	1.4786	6.4426	8.5527	9.1594	9.8809	10.7777	4.0663;
-0.0002	0.29	0.7364	3.7257	4.6952	5.0971	5.57	6.3597	3.0003;
1.9663	0.4678	0.4981	0.5783	0.549	0.5565	0.5637	0.5901	0.7378;
0.2966	0.3011	0.295	0.2658	0.3711	0.3814	0.4245	0.3793	-1.2536;
-0.0292	0.5531	1.3313	5.5525	7.9164	8.7014	9.3596	10.3076	3.832;
-0.023	0.242	0.6264	3.0118	4.2753	4.7378	5.2039	6.0424	2.7939;
0.787	0.4375	0.4705	0.5424	0.5401	0.5445	0.556	0.5862	0.7291;
0.2845	0.3062	0.2959	0.213	0.3556	0.3813	0.4158	0.4182	-1.2058;
0.0027	0.5215	1.2005	5.2407	7.2245	7.8964	8.6652	9.3737	3.6004;
0.0037	0.2172	0.5194	2.7472	3.675	4.096	4.6013	5.3534	2.5415;
1.3613	0.4164	0.4327	0.5242	0.5087	0.5187	0.531	0.5711	0.7059;
0.2868	0.2984	0.3035	0.1714	0.3074	0.2816	0.4045	0.4315	-1.1809;
0.0032	0.4744	1.0469	4.7343	6.759	7.2923	7.7609	8.5337	3.2481;
0.0054	0.179	0.3915	2.2943	3.2371	3.5137	3.8759	4.6227	2.1779;
1.7111	0.3774	0.3739	0.4846	0.4789	0.4818	0.4994	0.5417	0.6705;
0.2865	0.2988	0.3125	0.2126	0.3141	0.3044	0.3788	0.4087	-1.2033;
0.0065	0.4291	0.9333	4.0827	6.8615	7.3098	7.8867	8.5997	3.1052;
0.0094	0.1405	0.2985	1.7559	3.3187	3.5934	3.978	4.6746	2.0867;
1.435	0.3275	0.3198	0.4301	0.4837	0.4916	0.5044	0.5436	0.672
];

%================= 数据拆分 =================
Cx_fr  = flipud(z_f(1:4:end, :));
Cn_fr  = flipud(z_f(2:4:end, :));
Cm_fr  = flipud(z_f(3:4:end, :));
Xcp_fr = flipud(z_f(4:4:end, :));

Cx_rr  = z_r(1:4:end, :);
Cn_rr  = z_r(2:4:end, :);
Cm_rr  = z_r(3:4:end, :);
Xcp_rr = z_r(4:4:end, :);

%% 数据插值结果

%================= 二维插值 =================
Cx_fr_  = interp2(x, y, Cx_fr,  alpha, Forward, 'spline');
Cn_fr_  = interp2(x, y, Cn_fr,  alpha, Forward, 'spline');
Cm_fr_  = interp2(x, y, Cm_fr,  alpha, Forward, 'spline');
Xcp_fr_ = interp2(x, y, Xcp_fr, alpha, Forward, 'spline');

Cx_rr_  = interp2(x, y, Cx_rr,  alpha, Rudder, 'spline');
Cn_rr_  = interp2(x, y, Cn_rr,  alpha, Rudder, 'spline');
Cm_rr_  = interp2(x, y, Cm_rr,  alpha, Rudder, 'spline');
Xcp_rr_ = interp2(x, y, Xcp_rr, alpha, Rudder, 'spline');

%================= 合成 =================
Cx  = Cx_fr_ + Cx_rr_;
Cn  = Cn_fr_ + Cn_rr_;
Cm  = Cm_fr_ + Cm_rr_;

if (Cn_fr_ + Cn_rr_) ~= 0
    Xcp = (Cn_fr_*Xcp_fr_ + Cn_rr_*Xcp_rr_) / (Cn_fr_ + Cn_rr_);
else
    Xcp = 0;
end

end

== matlab function Rocketmodel/控制分配模块/1 ==
  data: Servo output; F_d input; M_d input; alpha input; Engine output; Forward output; Rudder output; u_opt output; V input
function [Servo, Engine, Forward, Rudder, u_opt] = allocation_opt(F_d, M_d, alpha, V)
% 优化分配模块（改进版）
% 功能: 根据期望力和期望力矩，计算发动机舵机、推力百分比和前后舵角
%
% 输入:
%   F_d    3x1 期望力向量 [N]
%   M_d    3x1 期望力矩向量 [N*m]
%   alpha  当前攻角 [rad]
%   V   落点系速度向量 [m/s]
%
% 输出:
%   Servo  6x1 三台发动机六个舵机角 [rad]
%   Engine 3x1 三台发动机推力百分比 [0~1]
%   Forward 前舵角 [rad]
%   Rudder  后舵角 [rad]
%   u_opt   11x1 优化器解向量

% 
% 
% F_d= [10000 20000 0];
% M_d=[0 0 140000];
% alpha=90/57.3;
% V=[-6 -80 0];

persistent u_prev  % 保存上一时刻优化解

% 第一次调用时初始化
if isempty(u_prev)
    u_prev = zeros(11,1);  % 必须先给值
end

% 初始猜测使用上一时刻解
u0 = u_prev;


%% ================== 内部参数定义 ==================
N_engine = 3;  % 发动机数量
Pe = 2.45e6;   % 单台发动机额定推力 [N]
r_engine = [ -15.2740  -15.2740  -15.2740;
               1.5      -0.75     -0.75;
               0        -1.299     1.299 ];  % 发动机在机体系下位置 [m]

rho = 1.2; % 空气密度 [kg/m^3]
S   = 63.617;     % 大气面积

%% ================== 初始猜测 ==================
% if isempty(u_prev)
%     u0 = zeros(11,1); % 首次调用初始化为0
% else
%     u0 = u_prev;       % 后续调用使用上一时刻解
% end

%% ================== 单变量上下界 ==================
lb = [-7.8*pi/180*ones(6,1); zeros(3,1); 0*pi/180; 0*pi/180];
ub = [ 7.8*pi/180*ones(6,1); ones(3,1);  180*pi/180;  180*pi/180];

%% ================== 合成摆角正八边形线性约束 ==================

Delta_max = 8*pi/180;  % 摆圆半径 8°
nServo = 6;            % 六个舵机
A = zeros(8*N_engine, nServo);
b = zeros(8*N_engine,1);

for i = 1:N_engine
    idx = 2*i-1; % 每台发动机的两个舵机索引
    A(8*(i-1)+1, idx)   = 1;     b(8*(i-1)+1)   = Delta_max;
    A(8*(i-1)+2, idx)   = -1;    b(8*(i-1)+2)   = Delta_max;
    A(8*(i-1)+3, idx+1) = 1;     b(8*(i-1)+3)   = Delta_max;
    A(8*(i-1)+4, idx+1) = -1;    b(8*(i-1)+4)   = Delta_max;
    A(8*(i-1)+5, idx)   = 1; A(8*(i-1)+5, idx+1) = 1;  b(8*(i-1)+5) = Delta_max*sqrt(2);
    A(8*(i-1)+6, idx)   = -1; A(8*(i-1)+6, idx+1) = -1; b(8*(i-1)+6) = Delta_max*sqrt(2);
    A(8*(i-1)+7, idx)   = 1; A(8*(i-1)+7, idx+1) = -1; b(8*(i-1)+7) = Delta_max*sqrt(2);
    A(8*(i-1)+8, idx)   = -1; A(8*(i-1)+8, idx+1) = 1; b(8*(i-1)+8) = Delta_max*sqrt(2);
end

nVar = 11; % 决策变量总数
A_full = zeros(size(A,1), nVar);
A_full(:,1:6) = A;  % 前 6 列是舵机约束
b_full = b;
 b=b_full;
 A = A_full;

%% ================== 气动力查表函数 ==================
aero = build_aero_lookup();

%% ================== 优化器调用 ==================
fun = @(u) cost_function(u, F_d, M_d, alpha, V, N_engine, Pe, r_engine, aero, rho, S);
% nonlcon = @(u) torque_balance_constraint(u, alpha, V, N_engine, Pe, r_engine, aero, rho, S);
options = optimoptions('fmincon','Display','none','Algorithm','sqp', ...
                       'MaxIterations',1000,'OptimalityTolerance',1e-4);
u_opt = fmincon(fun, u0, A, b, [], [], lb, ub, [], options);



% u_opt = fmincon(fun, u0, A, b, [], [], lb, ub, nonlcon, options);

% 保存本次解
u_prev = u_opt;

%% ================== 输出拆解 ==================
Servo   = u_opt(1:6);   % 六个伺服角
Engine  = u_opt(7:9);   % 三台发动机推力百分比
Forward = u_opt(10);    % 前舵角
Rudder  = u_opt(11);    % 后舵角
end


%% ---------------------- 子函数 ----------------------

function J = cost_function(u, F_d, M_d, alpha, V, N_engine, Pe, r_engine, aero, rho, S)
[F, M] = actuator_model(u, alpha, V, N_engine, Pe, r_engine, aero, rho, S);
J = norm(F - F_d)^2 + norm(M - M_d)^2;
end

function [F_total, M_total] = actuator_model(u, alpha, V, N_engine, Pe, r_engine, aero, rho, S)
delta_eng = u(1:6);   % 六个舵机角
P         = u(7:9);   % 三个发动机推力百分比
delta_f   = u(10);    % 前舵角
delta_r   = u(11);    % 后舵角

F_total = zeros(3,1);
M_total = zeros(3,1);

% ================== 三台发动机 ==================
for i = 1:N_engine
    delta_p = delta_eng(2*i-1);
    delta_y = delta_eng(2*i);
    D = [cos(delta_p)*cos(delta_y);
         -sin(delta_p);
         cos(delta_p)*sin(-delta_y)];
    F_i = P(i)*Pe * D;
    M_i = cross(r_engine(:,i), F_i);
    F_total = F_total + F_i;
    M_total = M_total + M_i;
end

% ================== 舵面气动力 ==================
Cx  = aero.Cx(delta_f, delta_r, alpha);
Cn  = aero.Cn(delta_f, delta_r, alpha);
Cm  = aero.Cm(delta_f, delta_r, alpha);
Xcp = aero.Xcp(delta_f, delta_r, alpha);


V = V; 
q = 0.5 * rho * norm(V)^2;

F_total = F_total + q*S*[-Cx; Cn; 0];
M_total = M_total + q*S*[0; 0; Cn*Xcp - Cm*47.8]; % L=47.8 m
end


function aero = build_aero_lookup()
x = [0,4,8,30,50,60,70,90,150]/57.3;
y = [0,20,40,60,80]/57.3;

% ----------- 前舵数据 -----------------
z_f = [0.2983	0.3105	0.3109	0.34	0.3102	0.36	0.3968	0.3115	-1.178;
0.0333	0.6536	1.442	5.3229	7.9765	8.5087	9.1668	9.894	3.4019;
0.0004	0.3464	0.8089	3.1887	4.5519	4.9497	5.3774	6.0923	2.8019;
0.0126	0.53	0.5609	0.599	0.5707	0.5817	0.5866	0.6158	0.8236;
0.2965	0.3117	0.3068	0.3731	0.3353	0.3577	0.4056	0.3175	-1.1556;
0.0433	0.6561	1.4587	5.4398	7.9116	8.4858	9.1227	9.8364	3.4092;
-0.0002	0.3129	0.7542	3.1904	4.5143	4.9434	5.3699	6.0813	2.8162;
-0.0044	0.4769	0.517	0.5865	0.5706	0.5826	0.5886	0.6182	0.8261;
0.2922	0.3164	0.3073	0.3742	0.3142	0.3435	0.3922	0.3478	-1.1666;
0.0595	0.6854	1.5233	5.6129	8.1435	8.7701	9.4561	10.1558	3.6688;
0.0169	0.3286	0.7791	3.2016	4.5616	4.985	5.4273	6.1567	2.9435;
0.2844	0.4794	0.5114	0.5704	0.5602	0.5684	0.5739	0.6062	0.8023;
0.2862	0.3039	0.2954	0.3019	0.3771	0.3267	0.4269	0.3565	-1.1929;
0.0006	0.6651	1.5116	6.0214	8.2621	9.098	9.5941	10.405	3.7881;
-0.0185	0.3289	0.7783	3.4086	4.5714	5.0651	5.4516	6.2152	2.9431;
0	0.4945	0.5149	0.5661	0.5533	0.5567	0.5682	0.5973	0.7769;
0.242	0.2554	0.2475	0.2483	0.3807	0.3942	0.4246	0.3628	-1.1474;
-0.0001	0.6199	1.4786	6.4426	8.5527	9.1594	9.8809	10.7777	4.0663;
-0.0002	0.29	0.7364	3.7257	4.6952	5.0971	5.57	6.3597	3.0003;
1.9663	0.4678	0.4981	0.5783	0.549	0.5565	0.5637	0.5901	0.7378;
];

% ----------- 后舵数据 -----------------
z_r = [0.242	0.2554	0.2475	0.2483	0.3807	0.3942	0.4246	0.3628	-1.1474;
-0.0001	0.6199	1.4786	6.4426	8.5527	9.1594	9.8809	10.7777	4.0663;
-0.0002	0.29	0.7364	3.7257	4.6952	5.0971	5.57	6.3597	3.0003;
1.9663	0.4678	0.4981	0.5783	0.549	0.5565	0.5637	0.5901	0.7378;
0.2966	0.3011	0.295	0.2658	0.3711	0.3814	0.4245	0.3793	-1.2536;
-0.0292	0.5531	1.3313	5.5525	7.9164	8.7014	9.3596	10.3076	3.832;
-0.023	0.242	0.6264	3.0118	4.2753	4.7378	5.2039	6.0424	2.7939;
0.787	0.4375	0.4705	0.5424	0.5401	0.5445	0.556	0.5862	0.7291;
0.2845	0.3062	0.2959	0.213	0.3556	0.3813	0.4158	0.4182	-1.2058;
0.0027	0.5215	1.2005	5.2407	7.2245	7.8964	8.6652	9.3737	3.6004;
0.0037	0.2172	0.5194	2.7472	3.675	4.096	4.6013	5.3534	2.5415;
1.3613	0.4164	0.4327	0.5242	0.5087	0.5187	0.531	0.5711	0.7059;
0.2868	0.2984	0.3035	0.1714	0.3074	0.2816	0.4045	0.4315	-1.1809;
0.0032	0.4744	1.0469	4.7343	6.759	7.2923	7.7609	8.5337	3.2481;
0.0054	0.179	0.3915	2.2943	3.2371	3.5137	3.8759	4.6227	2.1779;
1.7111	0.3774	0.3739	0.4846	0.4789	0.4818	0.4994	0.5417	0.6705;
0.2865	0.2988	0.3125	0.2126	0.3141	0.3044	0.3788	0.4087	-1.2033;
0.0065	0.4291	0.9333	4.0827	6.8615	7.3098	7.8867	8.5997	3.1052;
0.0094	0.1405	0.2985	1.7559	3.3187	3.5934	3.978	4.6746	2.0867;
1.435	0.3275	0.3198	0.4301	0.4837	0.4916	0.5044	0.5436	0.672
];

% 数据拆分
Cx_fr  = flipud(z_f(1:4:end, :));
Cn_fr  = flipud(z_f(2:4:end, :));
Cm_fr  = flipud(z_f(3:4:end, :));
Xcp_fr = flipud(z_f(4:4:end, :));

Cx_rr  = z_r(1:4:end, :);
Cn_rr  = z_r(2:4:end, :);
Cm_rr  = z_r(3:4:end, :);
Xcp_rr = z_r(4:4:end, :);

% 构建函数句柄
aero.Cx = @(Forward,Rudder,alpha) ...
    interp2(x, y, Cx_fr, alpha, Forward, 'spline') + ...
    interp2(x, y, Cx_rr, alpha, Rudder, 'spline');
aero.Cn = @(Forward,Rudder,alpha) ...
    interp2(x, y, Cn_fr, alpha, Forward, 'spline') + ...
    interp2(x, y, Cn_rr, alpha, Rudder, 'spline');
aero.Cm = @(Forward,Rudder,alpha) ...
    interp2(x, y, Cm_fr, alpha, Forward, 'spline') + ...
    interp2(x, y, Cm_rr, alpha, Rudder, 'spline');
aero.Xcp = @(Forward,Rudder,alpha) ...
    ((interp2(x, y, Cn_fr, alpha, Forward, 'spline').*interp2(x, y, Xcp_fr, alpha, Forward, 'spline')) + ...
     (interp2(x, y, Cn_rr, alpha, Rudder, 'spline').*interp2(x, y, Xcp_rr, alpha, Rudder, 'spline'))) ./ ...
    (interp2(x, y, Cn_fr, alpha, Forward, 'spline') + interp2(x, y, Cn_rr, alpha, Rudder, 'spline') + eps);
end


% function [c, ceq] = torque_balance_constraint(u, alpha, V, N_engine, Pe, r_engine, aero, rho, S)
%     [F, M] = actuator_model(u, alpha, V, N_engine, Pe, r_engine, aero, rho, S);
% 
%     c = [];  % 无不等式约束
%     ceq = M([1,2]); % Mx, My = 0 (滚转, 偏航)
% end

== matlab function Rocketmodel/火箭动力学与运动学模型/欧拉角转换方程 ==
  data: Euler_dot output; Omega input; Euler input
function Euler_dot  = fcn(Omega, Euler)

Euler_dot = NaN(3, 1);

Euler_dot(1) = Omega(1) + Omega(2) * tan(Euler(2)) * sin(Euler(1)) + Omega(3) * tan(Euler(2)) * cos(Euler(1));
Euler_dot(2) = Omega(2) * cos(Euler(1)) - Omega(3) * sin(Euler(1));
Euler_dot(3) = Omega(2) * sin(Euler(1)) / cos(Euler(2)) + Omega(3) * cos(Euler(1)) / cos(Euler(2));

== matlab function Rocketmodel/火箭动力学与运动学模型/绕质心动力学方程 ==
  data: Omega_dot output; Omega input; Mc input; Mp input
function Omega_dot   = fcn(Omega, Mc, Mp)


Jx = 194500;
Jy = 13280000;
Jz = 13280000;

Omega_dot = NaN(3, 1);


Omega_dot(1) = (Jz - Jy) / Jx * Omega(2) * Omega(3) + (Mc(1) + Mp(1)) / Jx; 
Omega_dot(2) = (Jx - Jz) / Jy * Omega(3) * Omega(1) + (Mc(2) + Mp(2)) / Jy; 
Omega_dot(3) = (Jy - Jx) / Jz * Omega(2) * Omega(1) + (Mc(3) + Mp(3)) / Jz;

== matlab function Rocketmodel/火箭动力学与运动学模型/质心位置方程 ==
  data: R_dot output; V input
function R_dot  = fcn(V)


R_dot = V;

== matlab function Rocketmodel/火箭动力学与运动学模型/质心运动方程 ==
  data: C_body_to_land input; C_ecef_to_land input; V_dot output; Fc input; Fp input; Fg input
function V_dot  = fcn(C_body_to_land, C_ecef_to_land, Fc, Fp, Fg)

%% 函数说明
%   落点系下火箭质心运动方程

%% 基本参数引入
% 火箭质量
M0 = 155975;

%% 火箭运动学方程
V_dot = NaN(3,1);

A = C_body_to_land * Fc + C_ecef_to_land * Fg + C_body_to_land * Fp;


V_dot(1) = A(1)/M0;
V_dot(2) = A(2)/M0;
V_dot(3) = A(3)/M0;



end

== matlab function Rocketmodel/火箭动力学与运动学模型/箭体系与落点系之间的旋转矩阵 ==
  data: C_land_to_body output; Euler input; C_body_to_land output
function [C_land_to_body, C_body_to_land] = fcn(Euler)

C_land_to_body = [cos(Euler(3)) * cos(Euler(2)), sin(Euler(3)) * cos(Euler(2)), - sin(Euler(2));
    - sin(Euler(3))*cos(Euler(1)) + cos(Euler(3))*sin(Euler(2))*sin(Euler(1)), cos(Euler(3))*cos(Euler(1)) + sin(Euler(3))*sin(Euler(2))*sin(Euler(1)), cos(Euler(2))*sin(Euler(1));
    sin(Euler(3))*sin(Euler(1)) + cos(Euler(3))*sin(Euler(2))*cos(Euler(1)), - cos(Euler(3))*sin(Euler(1)) + sin(Euler(3))*sin(Euler(2))*cos(Euler(1)), cos(Euler(2))*cos(Euler(1))];

C_body_to_land =  C_land_to_body'; 

end

== matlab function Rocketmodel/火箭动力学与运动学模型/落点系与地心地固系之间的旋转矩阵 ==
  data: C_land_to_ecef output; C_ecef_to_land output
function [C_land_to_ecef, C_ecef_to_land]  = fcn()

%%  旋转矩阵、平动向量等参数计算


%%  旋转矩阵、平动向量等参数计算

% 火箭质量

M0 = 155975;

% WGS-84参数

a = 6378137;  
f = 1/298.257223563;
e_2 =2*f - f^2;
b = a*(1 - f);
miu = 3.986004418e14;
J_2 = 1.08263e-3;

% 求落点系land原点在地心地固系ECEF下坐标 
 
L0 = 110.95; %  着陆点经纬高
B0 = 19.6; 
H0 = 0; 

N_B = a/sqrt(1 - e_2*(sind(B0))^2); 
R0_ecef = [(N_B + H0)*cosd(B0)*cosd(L0), (N_B + H0)*cosd(B0)*sind(L0), ((1-e_2)*N_B + H0)*sind(B0)]';


% 求落点系到局部东北天坐标系的旋转矩阵

A0 = 110.3; % 着陆方位角   注意rot函数正数代表顺时针旋转。耽误我好久，气死我了

C_land_to_enu = rotz(90-A0) * rotx(90); 


% 求局部东北天坐标系到地心地固坐标系的旋转矩阵

C_enu_to_ecef = rotz(90+L0)*rotx(90-B0); 

% 求落点系到地心地固系的旋转矩阵 

C_land_to_ecef = C_enu_to_ecef * C_land_to_enu; 

% 求发射系到地心地固系的转换公式 旋转+平动

C_land_to_ecef  = C_land_to_ecef; 
R0_ecef = R0_ecef;


C_ecef_to_land = C_land_to_ecef;

end

== matlab function Rocketmodel/火箭动力学与运动学模型/攻角计算方程 ==
  data: alpha output; V input; C_land_to_body input
function alpha   = fcn(V, C_land_to_body)



Vb = C_land_to_body * V;

if Vb(1) == 0
    alpha = 90/57.3;
else
    alpha = abs(atan2(Vb(2), Vb(1)));
end
